simulink model "gm_sla_VHT_HDL_fil"  (R2015b)
settings: Solver=FixedStepDiscrete  SolverMode=SingleTasking  StartTime=0.0  StopTime=320*240*102  RelTol=1e-3
PreLoadFcn:
  | H = fspecial('unsharp')
undefined symbols (not defined in the file or in its folder): gray
libraries: visionsinks x4, visionconversions x2, visionfilter x1, simulink x1, fillib x1, visionhdlio x1, dspmtrx3 x1, dspvision x1
settings Model: SimulationMode=accelerator  Creator=yutengz  LastModifiedBy=amatsumo
settings DataIOCC: SaveFormat=Array
settings OptimizationCC: BlockReduction=off  BooleanDataType=off  ConditionallyExecuteInputs=off
settings DebuggingCC: SaveWithParameterizedLinksMsg=none  UnderspecifiedInitializationDetection=Classic  MergeDetectMultiDrivingBlocksExec=none  SignalResolutionControl=TryResolveAllWithWarning  InheritedTsInSrcMsg=none
settings HardwareCC: ProdBitPerPointer=32  ProdLargestAtomicFloat=None  ProdIntDivRoundTo=Undefined  ProdEndianess=Unspecified  ProdWordSize=32  ProdHWDeviceType=32-bit Generic  TargetUnknown=on
settings GRTTargetCC: GeneratePreprocessorConditionals=Disable all
settings ConfigComp: CovModelRefEnable=Off  CovSFcnEnable=off

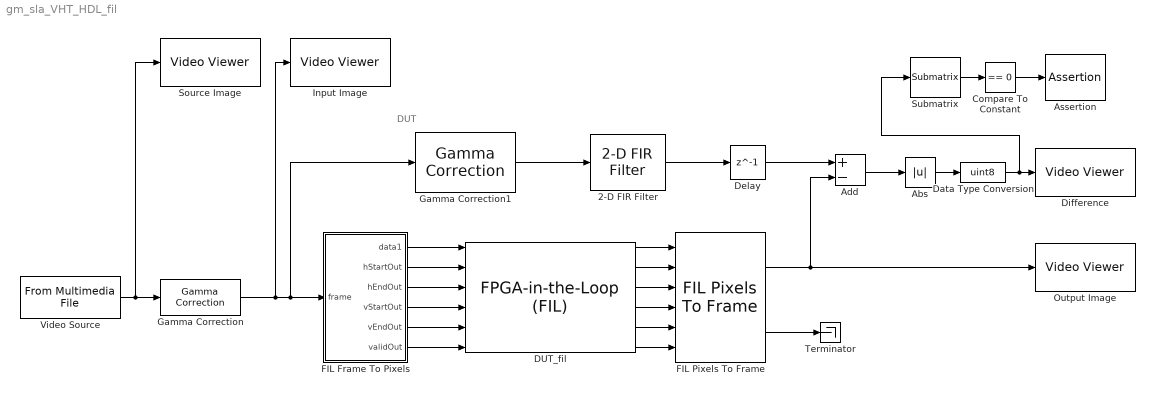
== system gm_sla_VHT_HDL_fil ==
  note: DUT
  2-D FIR Filter : visionfilter/2-D FIR Filter  separable=off  filtSrc=Specify via dialog  filterMtrx=H  verticalFilter=[4 0]  horizontalFilter=[4 0]  outSize=Same as input port I  padType=Constant  padSrc=Specify via dialog  padVal=0  method=Convolution  firstCoeffMode=Binary point scaling  firstCoeffWordLength=8  firstCoeffFracLength=4  firstCoeffSignedness=Signed  firstCoeffDataTypeStr=fixdt(1,8,4)  firstCoeffLastDataTypeStr=fixdt(1,8,4)  firstCoeffMin=[]  firstCoeffMax=[]  outputSignedness=Auto  outputMin=[]  outputMax=[]  accumDataTypeStr=Inherit: Same as product output  accumLastDataTypeStr=Inherit: Same as product output  prodOutputMode=Binary point scaling  prodOutputWordLength=32  prodOutputFracLength=10  prodOutputDataTypeStr=fixdt([],32,10)  prodOutputLastDataTypeStr=fixdt([],32,10)  roundingMode=Floor  overflowMode=on
  Abs : Abs
  Add : Sum  Inputs=+-  OutDataTypeStr=int16
  Assertion : Assertion
  Compare To Constant : simulink/Logic and Bit Operations/Compare To Constant  relop===  const=0  OutDataTypeStr=boolean
  DUT_fil : fillib/FPGA-in-the-Loop (FIL)  ForceInterfaceUpdate=0.91338
      settings: AttributesFormatString=IP Address: 192.168.1.10
  Data Type Conversion : DataTypeConversion  OutDataTypeStr=uint8
  Delay : Delay  DelayLength=1  InputProcessing=Inherited
  Difference : visionsinks/Video Viewer  inputType=Obsolete7b  imagePorts=One multidimensional signal  useColorMap=off  colormapValue=gray(256)  specRange=off  minInputVal=0  maxInputVal=255  FigPos=[1057 383 334 275]  AxisZoom=on  trueSizedOnce=off  OpenAtMdlStart=on  DefaultConfigurationName=vipscopes.VideoViewerScopeCfg
  FIL Frame To Pixels : Subsystem  mask(FIL Frame To Pixels){NumComponents=1, OutputVectorFormat=Frame, VideoFormat=240p, ActivePixelsPerLine=32, ActiveVideoLines=18, TotalPixelsPerLine=42, TotalVideoLines=28, StartingActiveLine=6, FrontPorch=5, SampleTime=0}
      mask prompts: NumComponents "Number of components:"; OutputVectorFormat "Output vector format:"; VideoFormat "Video format:"; ActivePixelsPerLine "Active pixels per line:"; ActiveVideoLines "Active video lines:"; TotalPixelsPerLine "Total pixels per line:"; TotalVideoLines "Total video lines:"; StartingActiveLine "Starting active line:"; FrontPorch "Front porch:"; SampleTime "Sample Time"
      mask init:
      | visionhdl.internal.CommonSets.gatewayInFIL(gcb, 'init');
      mask TypeOptions OutputVectorFormat: Pixel | Line | Frame
      mask TypeOptions VideoFormat: hf2p/VideoFormat
      mask Callback VideoFormat: visionhdl.internal.CommonSets.gatewayInFIL(gcb, 'videoformat');
      mask TypeOptions ActivePixelsPerLine: hf2p/ActivePixelsPerLine
      mask TypeOptions ActiveVideoLines: hf2p/ActiveVideoLines
      mask TypeOptions TotalPixelsPerLine: hf2p/TotalPixelsPerLine
      mask TypeOptions TotalVideoLines: hf2p/TotalVideoLines
      mask TypeOptions StartingActiveLine: hf2p/StartingActiveLine
      mask TypeOptions FrontPorch: hf2p/FrontPorch
      mask DialogControl InfoGroup Prompt: Video Format Parameters
      mask Display: disp('FIL\nFrame To Pixels');
  FIL Pixels To Frame : visionhdlio/FIL Pixels To Frame  NumComponents=1  InputVectorFormat=Frame  VideoFormat=240p  ActivePixelsPerLine=32  ActiveVideoLines=18  TotalPixelsPerLine=42  TotalVideoLines=28
  Gamma Correction : visionconversions/Gamma Correction  operation=De-gamma  gamma=2.2  linearSegment=on  breakPoint=0.018
  Gamma Correction1 : visionconversions/Gamma Correction  operation=Gamma  gamma=2.2  linearSegment=on  breakPoint=0.018
  Input Image : visionsinks/Video Viewer  inputType=Obsolete7b  imagePorts=One multidimensional signal  useColorMap=off  colormapValue=gray(256)  specRange=off  minInputVal=0  maxInputVal=255  FigPos=[366 381 334 275]  AxisZoom=on  trueSizedOnce=off  OpenAtMdlStart=on  DefaultConfigurationName=vipscopes.VideoViewerScopeCfg
  Output Image : visionsinks/Video Viewer  inputType=Obsolete7b  imagePorts=One multidimensional signal  useColorMap=off  colormapValue=gray(256)  specRange=off  minInputVal=0  maxInputVal=255  FigPos=[709 384 334 275]  AxisZoom=on  trueSizedOnce=off  OpenAtMdlStart=on  DefaultConfigurationName=vipscopes.VideoViewerScopeCfg
  Source Image : visionsinks/Video Viewer  inputType=Obsolete7b  imagePorts=One multidimensional signal  useColorMap=off  colormapValue=gray(256)  specRange=off  minInputVal=0  maxInputVal=255  FigPos=[21 379 334 275]  AxisZoom=on  trueSizedOnce=off  OpenAtMdlStart=on  DefaultConfigurationName=vipscopes.VideoViewerScopeCfg
  Submatrix : dspmtrx3/Submatrix  RowSpan=Range of rows  RowStartMode=Index  RowStartIndex=2  RowEndMode=Index  RowEndIndex=239  ColSpan=Range of columns  ColStartMode=Index  ColStartIndex=2  ColEndMode=Index  ColEndIndex=319
  Terminator : Terminator
  Video Source : dspvision/From Multimedia File  inputFilename=rhinos.avi  loop=on  numPlays=inf  outputStreams=Video only  videoDataType=uint8  audioDataType=int16  inheritSampleTime=off  userDefinedSampleTime=402*324  noAudioOutput=off  isIntensityVideo=off  fourcc=Intensity  colorVideoFormat=One multidimensional signal  outputEOF=off  dataOrg=Column-major  audioFrameSize=1024  computeAudioFrameSize=off  outSamplingMode=Sample based
  wires:
  Video Source/1 -> Source Image/1, Gamma Correction/1
  FIL Pixels To Frame/1 -> Output Image/1, Add/2
  FIL Pixels To Frame/2 -> Terminator/1
  2-D FIR Filter/1 -> Delay/1
  Gamma Correction/1 -> FIL Frame To Pixels/1(frame), Gamma Correction1/1, Input Image/1
  Gamma Correction1/1 -> 2-D FIR Filter/1
  Add/1 -> Abs/1
  Abs/1 -> Data Type Conversion/1
  Delay/1 -> Add/1
  DUT_fil/1 -> FIL Pixels To Frame/1
  DUT_fil/2 -> FIL Pixels To Frame/2
  DUT_fil/3 -> FIL Pixels To Frame/3
  DUT_fil/4 -> FIL Pixels To Frame/4
  DUT_fil/5 -> FIL Pixels To Frame/5
  DUT_fil/6 -> FIL Pixels To Frame/6
  FIL Frame To Pixels/1(data1) -> DUT_fil/1
  FIL Frame To Pixels/2(hStartOut) -> DUT_fil/2
  FIL Frame To Pixels/3(hEndOut) -> DUT_fil/3
  FIL Frame To Pixels/4(vStartOut) -> DUT_fil/4
  FIL Frame To Pixels/5(vEndOut) -> DUT_fil/5
  FIL Frame To Pixels/6(validOut) -> DUT_fil/6
  Data Type Conversion/1 -> Submatrix/1, Difference/1
  Submatrix/1 -> Compare To Constant/1
  Compare To Constant/1 -> Assertion/1

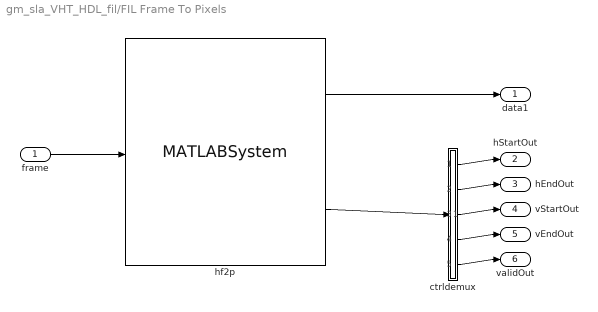
== system gm_sla_VHT_HDL_fil/FIL Frame To Pixels ==
  frame : Inport
  ctrldemux : Subsystem
  hf2p : MATLABSystem  System=visionhdl.internal.FrameToFrameOfPixels  NumComponents=1  VideoFormat=240p  ActivePixelsPerLine=ActivePixelsPerLine  ActiveVideoLines=ActiveVideoLines  TotalPixelsPerLine=TotalPixelsPerLine  TotalVideoLines=TotalVideoLines  StartingActiveLine=StartingActiveLine  FrontPorch=FrontPorch  SimulateUsing=Code generation
      mask Type: visionhdl.internal.FrameToFrameOfPixels
      mask Display:
      | disp('FrameToFrameOfPixels');
      | port_label('input',1,'matrix');
      | port_label('output',1,'pixel');
      | port_label('output',2,'ctrl');
  data1 : Outport
  hStartOut : Outport  Port=2
  hEndOut : Outport  Port=3
  vStartOut : Outport  Port=4
  vEndOut : Outport  Port=5
  validOut : Outport  Port=6
  wires:
  frame/1 -> hf2p/1
  ctrldemux/1(output1) -> hStartOut/1
  ctrldemux/2(output2) -> hEndOut/1
  ctrldemux/3(output3) -> vStartOut/1
  ctrldemux/4(output4) -> vEndOut/1
  ctrldemux/5(output5) -> validOut/1
  hf2p/1 -> data1/1
  hf2p/2 -> ctrldemux/1(In1)

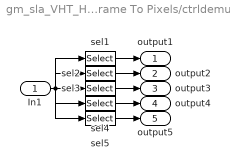
== system gm_sla_VHT_HDL_fil/FIL Frame To Pixels/ctrldemux ==
  In1 : Inport
  sel1 : Selector  NumberOfDimensions=2  InputPortWidth=3  IndexOptions=Select all,Index vector (dialog)  Indices=[1 5],1  OutputSizes=1
  sel2 : Selector  NumberOfDimensions=2  InputPortWidth=3  IndexOptions=Select all,Index vector (dialog)  Indices=[1 5],2  OutputSizes=1
  sel3 : Selector  NumberOfDimensions=2  InputPortWidth=3  IndexOptions=Select all,Index vector (dialog)  Indices=[1 5],3  OutputSizes=1
  sel4 : Selector  NumberOfDimensions=2  InputPortWidth=3  IndexOptions=Select all,Index vector (dialog)  Indices=[1 5],4  OutputSizes=1
  sel5 : Selector  NumberOfDimensions=2  InputPortWidth=3  IndexOptions=Select all,Index vector (dialog)  Indices=[1 5],5  OutputSizes=1
  output1 : Outport
  output2 : Outport  Port=2
  output3 : Outport  Port=3
  output4 : Outport  Port=4
  output5 : Outport  Port=5
  wires:
  In1/1 -> sel1/1, sel2/1, sel3/1, sel4/1, sel5/1
  sel1/1 -> output1/1
  sel2/1 -> output2/1
  sel3/1 -> output3/1
  sel4/1 -> output4/1
  sel5/1 -> output5/1
